simulink model "SinglePhaseInverter"  (R2021a)
settings: Solver=ode15s  StartTime=0.0  StopTime=0.1  FixedStep=1/fsw*PWM_Resolution  MaxStep=1/(4*fsw)  RelTol=1e-3  AbsTol=1e-3
PreLoadFcn:
  | Palam_SingleInverter;
undefined symbols (not defined in the file): DeadTime, fg, fsw, Initial_M, Kp, MaxDuty, MinDuty, Simple, Simscape, Ti, TimerCountMax, VinDC, VoutAC_rms
libraries: ee_lib x6, fl_lib x4, nesl_utility x4, slpidlib x1, eeGeneralControl x1, simulink x1
CloseFcn:
  | clear all
settings Model: Creator=ykamatan  LastModifiedBy=ykamatan
settings SolverCC: DaesscMode=Robust  ZeroCrossControl=EnableAll  ZeroCrossAlgorithm=Adaptive  AlgebraicLoopSolver=TrustRegion  ODENIntegrationMethod=ode1
settings DebuggingCC: SymbolicDimsDataTypeCodeGenerationDiagnostic=none  SFMachineParentedDataDiag=warning
settings SFSimCC: CustomCodeUndefinedFunction=UseInterfaceOnly
settings SimscapeCC: SimscapeLogType=local  SimscapeLogSimulationStatistics=on  SimscapeLogToSDI=on  SimscapeLogLimitData=off  SimscapeLogDataHistory=10000

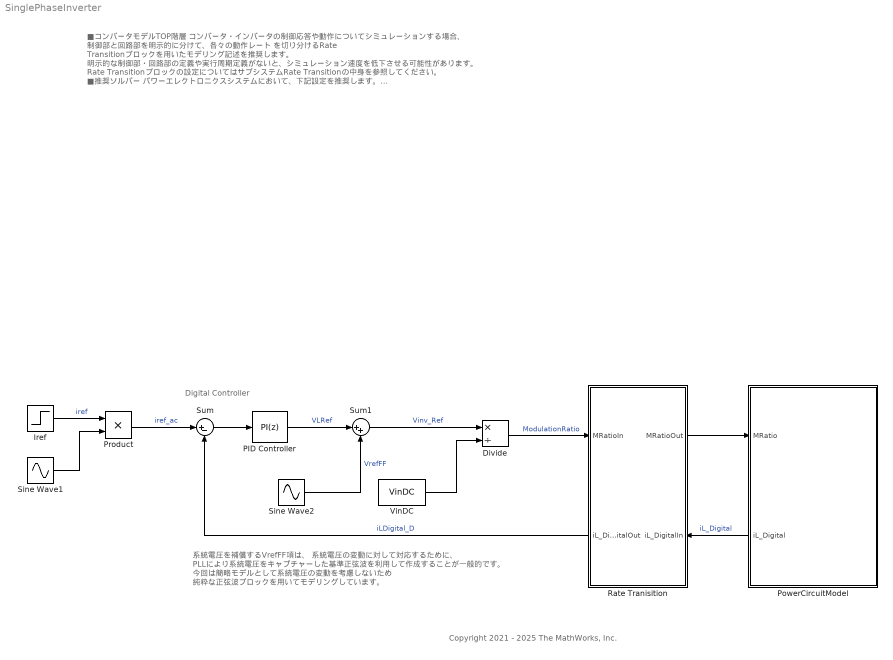
== system SinglePhaseInverter ==
  note: 系統電圧を補償するVrefFF項は、
      | 系統電圧の変動に対して対応するために、
      | PLLにより系統電圧をキャプチャーした基準正弦波を利用して作成することが一般的です。
      |
      | 今回は簡略モデルとして系統電圧の変動を考慮しないため
      | 純粋な正弦波ブロックを用いてモデリングしています。
  note: ■コンバータモデルTOP階層
      | コンバータ・インバータの制御応答や動作についてシミュレーションする場合、
      | 制御部と回路部を明示的に分けて、各々の動作レート を切り分けるRate Transitionブロックを用いたモデリング記述を推奨します。
      | 明示的な制御部・回路部の定義や実行周期定義がないと、シミュレーション速度を低下させる可能性があります。
      | Rate Transitionブロックの設定についてはサブシステムRate Transitionの中身を参照してください。
      |
      | ■推奨ソルバー
      | パワーエレクトロニクスシステムにおいて、下記設定を推奨します。
      | 最大ステップサイズに指定で用いている変数fswはスイッチング周波数です。
      | 最大ステップサイズを指定することで、可変ステップソルバがステップ数を長くしすぎることで、
      | Duｔｙパルス幅が指定周期に逐次更新されず、ずっとターンオンもしくはターンオンでシミュレーションが進行する現象が発生しなくなります。
  note: Digital Controller
  note: Copyright 2021 - 2025 The MathWorks, Inc.
  Divide : Product  Inputs=*/
  Iref : Step  Time=0.052  Before=5  After=10  SampleTime=1/fsw
  PID Controller : slpidlib/PID Controller  Controller=PI  Form=Parallel  TimeDomain=Discrete-time  UseExternalTs=off  SampleTime=1/fsw  IntegratorMethod=Forward Euler  FilterMethod=Forward Euler  ControllerParametersSource=internal  P=Kp  I=Ti  D=0  UseFilter=on  N=100  TunerSelectOption=Transfer Function Based (PID Tuner App)  InitialConditionSource=internal  InitialConditionForIntegrator=0  InitialConditionForFilter=0  DifferentiatorICPrevScaledInput=0  ExternalReset=none  TrackingMode=off  Kt=1  LimitOutput=off  SatLimitsSource=internal  UpperSaturationLimit=inf  LowerSaturationLimit=-inf  LinearizeAsGain=on  AntiWindupMode=none  Kb=1  POutMin=[]  POutMax=[]  IOutMin=[]  IOutMax=[]  DOutMin=[]  DOutMax=[]  NOutMin=[]  NOutMax=[]  SumOutMin=[]  SumOutMax=[]  SaturationOutMin=[]  SaturationOutMax=[]  PParamMin=[]  PParamMax=[]  IParamMin=[]  IParamMax=[]  DParamMin=[]  DParamMax=[]  NParamMin=[]  NParamMax=[]  KbParamMin=[]  KbParamMax=[]  KtParamMin=[]  KtParamMax=[]  KbOutMin=[]  KbOutMax=[]  KtOutMin=[]  KtOutMax=[]  IntegratorOutMin=[]  IntegratorOutMax=[]  FilterOutMin=[]  FilterOutMax=[]  SumI1OutMin=[]  SumI1OutMax=[]  SumI2OutMin=[]  SumI2OutMax=[]  SumI3OutMin=[]  SumI3OutMax=[]  SumI4OutMin=[]  SumI4OutMax=[]  SumDOutMin=[]  SumDOutMax=[]  DifferentiatorOutMin=[]  DifferentiatorOutMax=[]  FilterDiffOutCoefMin=[]  FilterDiffOutCoefMax=[]  ReciprocalOutMin=[]  ReciprocalOutMax=[]  SumDenOutMin=[]  SumDenOutMax=[]  SumNumOutMin=[]  SumNumOutMax=[]  DivideOutMin=[]  DivideOutMax=[]  UdiffTsProdOutMin=[]  UdiffTsProdOutMax=[]  NTsProdOutMin=[]  NTsProdOutMax=[]  UintegralTsProdOutMin=[]  UintegralTsProdOutMax=[]  UngainTsProdOutMin=[]  UngainTsProdOutMax=[]  IntegratorContinuousStateAttributes=''  IntegratorStateMustResolveToSignalObject=off  IntegratorRTWStateStorageClass=Auto  FilterContinuousStateAttributes=''  FilterStateMustResolveToSignalObject=off  FilterRTWStateStorageClass=Auto  ParallelPVariant=InternalParameters  IdealPVariant=Disabled  IVariant=InternalParameters  DVariant=Disabled  IntegratorVariant=Discrete  SatVariant=Disabled  AWVariant=Passthrough  PCopyVariant=Disabled  TRVariant=Disabled  FdbkBlocksVariant=Forward  IdealPFdbkVariant=Disabled  SatFdbkVariant=Disabled  DerivativeFilterVariant=Disabled  NVariant=Disabled  NCopyVariant=Disabled_SignalSpec  FilterICVariant=Disabled  IntegratorICVariant=InternalICs  ExternalResetVariant=Disabled  TRSumVariant=Passthrough  SumFdbkVariant=Disabled  SumVariant=Sum_PI  TsampFilterVariant=InternalTs  TsampNgainVariant=Passthrough  TsampIntegralVariant=Passthrough  ExternalSaturationOutDataTypeStr=Inherit: Same as second input
  PowerCircuitModel : Subsystem  VariantControl=Simulink+Simscape(Simple)
      settings: PortSchema="{\"entries\":[{\"content\":{\"sides\":[{\"content\":{\"connectorIds\":[\"In1\",\"Out1\"]},\"type\":\"ConnectorPlacement.EquallySpacedRectSide\",\"uuid\":\"190e0dea-1aa3-4142-a809-3b45efebbd06\"},{\"content\":{\"connectorIds\":[],\"side\":\"RIGHT\"},\"type\":\"ConnectorPlacement.EquallySpacedRectSide\",\"uuid\":\"b937fb0f-45e6-40ea-b2c8-56a8d22a3e17\"},{\"content\":{\"connectorIds\":[],\"side\":\"TOP\"},\"type\":\"ConnectorPlacement.EquallySpacedRectSide\",\"uuid\":\"78929584-fb1e-4361-895f-78605ee7c8f8\"}]},\"type\":\"ConnectorPlacement.EquallySpacedConnector\",\"uuid\":\"8246c905-c24d-44c3-959b-73866b615c12\"}],\"packageUris\":[\"http://schema.mathworks.com/mf0/Connector/R2020b\"],\"version\":\"1.0\"}"
  Product : Product
  "Rate Tranisition " : Subsystem
      settings: PortSchema="{\"entries\":[{\"content\":{\"sides\":[{\"content\":{\"connectorIds\":[\"In1\",\"Out2\"]},\"type\":\"ConnectorPlacement.EquallySpacedRectSide\",\"uuid\":\"82fdd683-de0b-47f1-9418-2e57132da0d0\"},{\"content\":{\"connectorIds\":[\"Out1\",\"In2\"],\"side\":\"RIGHT\"},\"type\":\"ConnectorPlacement.EquallySpacedRectSide\",\"uuid\":\"07812756-bbdf-4a3e-b825-c2cce10242a3\"},{\"content\":{\"connectorIds\":[],\"side\":\"TOP\"},\"type\":\"ConnectorPlacement.EquallySpacedRectSide\",\"uuid\":\"2a69d2b0-ad53-492d-9041-fc24e9d8466e\"}]},\"type\":\"ConnectorPlacement.EquallySpacedConnector\",\"uuid\":\"5e8493d4-adb1-45a0-b631-53482b8c22b1\"}],\"packageUris\":[\"http://schema.mathworks.com/mf0/Connector/R2020b\"],\"version\":\"1.0\"}"
  Sine Wave1 : Sin  Frequency=2*pi*fg  SampleTime=1/fsw
  Sine Wave2 : Sin  Amplitude=VoutAC_rms*sqrt(2)  Frequency=2*pi*fg  SampleTime=1/fsw
  Sum : Sum  Inputs=|+-
  Sum1 : Sum  Inputs=|++
  VinDC : Constant  Value=VinDC
  wires:
  PID Controller/1 -> Sum1/1  "VLRef"
  Sum/1 -> PID Controller/1
  Sum1/1 -> Divide/1  "Vinv_Ref"
  VinDC/1 -> Divide/2
  Product/1 -> Sum/1  "iref_ac"
  Divide/1 -> "Rate Tranisition "/1(MRatioIn)  "ModulationRatio"
  PowerCircuitModel/1(iL_Digital) -> "Rate Tranisition "/2(iL_DigitalIn)  "iL_Digital"
  "Rate Tranisition "/2(iL_DigitalOut) -> Sum/2  "iLDigital_D"
  "Rate Tranisition "/1(MRatioOut) -> PowerCircuitModel/1(MRatio)
  Iref/1 -> Product/1  "iref"
  Sine Wave1/1 -> Product/2
  Sine Wave2/1 -> Sum1/2  "VrefFF"

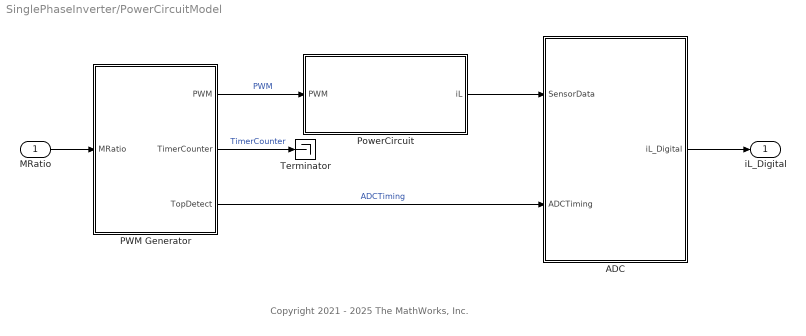
== system SinglePhaseInverter/PowerCircuitModel ==
  note: Copyright 2021 - 2025 The MathWorks, Inc.
  MRatio : Inport
  ADC : Subsystem
  PWM Generator : Subsystem
  PowerCircuit : Subsystem
  Terminator : Terminator
  iL_Digital : Outport
  wires:
  PowerCircuit/1(iL) -> ADC/1(SensorData)
  PWM Generator/1(PWM) -> PowerCircuit/1(PWM)  "PWM"
  PWM Generator/2(TimerCounter) -> Terminator/1  "TimerCounter"
  ADC/1(iL_Digital) -> iL_Digital/1
  MRatio/1 -> PWM Generator/1(MRatio)
  PWM Generator/3(TopDetect) -> ADC/2(ADCTiming)  "ADCTiming"

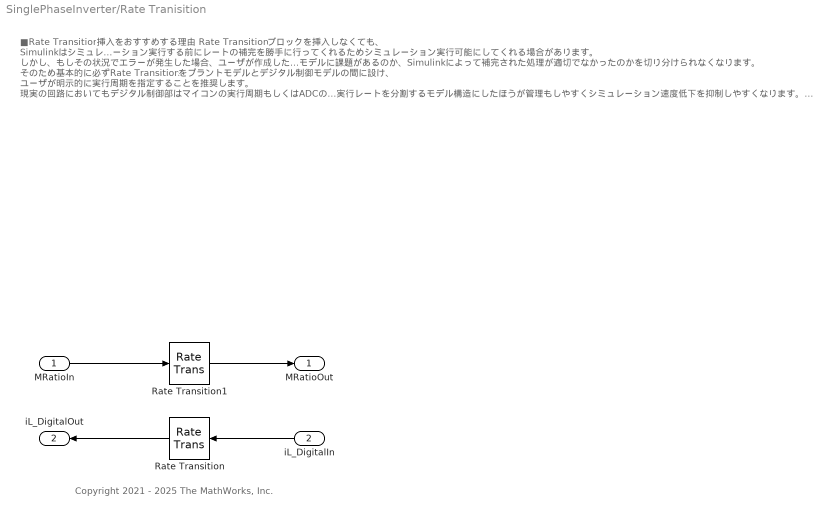
== system SinglePhaseInverter/Rate Tranisition  ==
  note: ■Rate Transition挿入をおすすめする理由
      | Rate Transitionブロックを挿入しなくても、
      | Simulinkはシミュレーション実行する前にレートの補完を勝手に行ってくれるためシミュレーション実行可能にしてくれる場合があります。
      |
      | しかし、もしその状況でエラーが発生した場合、ユーザが作成したモデルに課題があるのか、Simulinkによって補完された処理が適切でなかったのかを切り分けられなくなります。
      |
      | そのため基本的に必ずRate Transitionをプラントモデルとデジタル制御モデルの間に設け、
      | ユーザが明示的に実行周期を指定することを推奨します。
      |
      | 現実の回路においてもデジタル制御部はマイコンの実行周期もしくはADCの変換タイミングをトリガーに周期的に処理を行うため、明示的に実行レートを分割するモデル構造にしたほうが管理もしやすくシミュレーション速度低下を抑制しやすくなります。
      |
      | ■Rate Transitionのブロックパラメータ設定方法
      | ・データ転送中の整合性を確保
      | ・確定的にデータ転送を確保（最大遅延）
      | のチェックを入れておくことで、想定される最大のサンプリング遅れでサンプル値を取得するようにシミュレーションが動作します。これにより代数ループ警告も回避することができます。
      | ただし、このモデルのサンプリングはデジタルControllerモデルの実行周期(Tcnt = 1/fsw）分だけ必ずサンプリング値が遅れて伝搬されるため、制御ループの伝達関数を解析した際のむだ時間遅れは常に最悪の e^-sTcntとなることに注意が必要です。
  note: Copyright 2021 - 2025 The MathWorks, Inc.
  MRatioIn : Inport
  iL_DigitalIn : Inport  Port=2
  Rate Transition : RateTransition  OutPortSampleTime=1/fsw
  Rate Transition1 : RateTransition  InitialCondition=Initial_M
  MRatioOut : Outport
  iL_DigitalOut : Outport  Port=2
  wires:
  Rate Transition/1 -> iL_DigitalOut/1
  MRatioIn/1 -> Rate Transition1/1
  Rate Transition1/1 -> MRatioOut/1
  iL_DigitalIn/1 -> Rate Transition/1

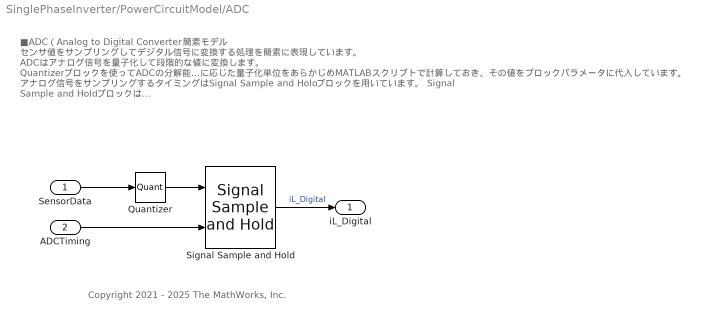
== system SinglePhaseInverter/PowerCircuitModel/ADC ==
  note: ■ADC（Analog to Digital Converter)簡素モデル
      | センサ値をサンプリングしてデジタル信号に変換する処理を簡素に表現しています。
      | ADCはアナログ信号を量子化して段階的な値に変換します。
      | Quantizerブロックを使ってADCの分解能に応じた量子化単位をあらかじめMATLABスクリプトで計算しておき、その値をブロックパラメータに代入しています。
      | アナログ信号をサンプリングするタイミングはSignal Sample and Holdブロックを用いています。
      | Signal Sample and Holdブロックは
      | Inにサンプリングしたい信号、Sにサンプリングタイミングを指定するパルス信号を入力することで、
      | そのタイミングでInの値をサンプリングし、それ以降次のパルスが入るまで値を保持します。
  note: Copyright 2021 - 2025 The MathWorks, Inc.
  SensorData : Inport
  ADCTiming : Inport  Port=2
  Quantizer : Quantizer  QuantizationInterval=QuantUnit
  Signal Sample and Hold : eeGeneralControl/Signal Sample and Hold  LabelModeActiveChoice=Discrete  x0=0  Ts=-1
      settings: SourceProductBaseCode=PS
  iL_Digital : Outport
  wires:
  Quantizer/1 -> Signal Sample and Hold/1
  Signal Sample and Hold/1 -> iL_Digital/1  "iL_Digital"
  ADCTiming/1 -> Signal Sample and Hold/2
  SensorData/1 -> Quantizer/1

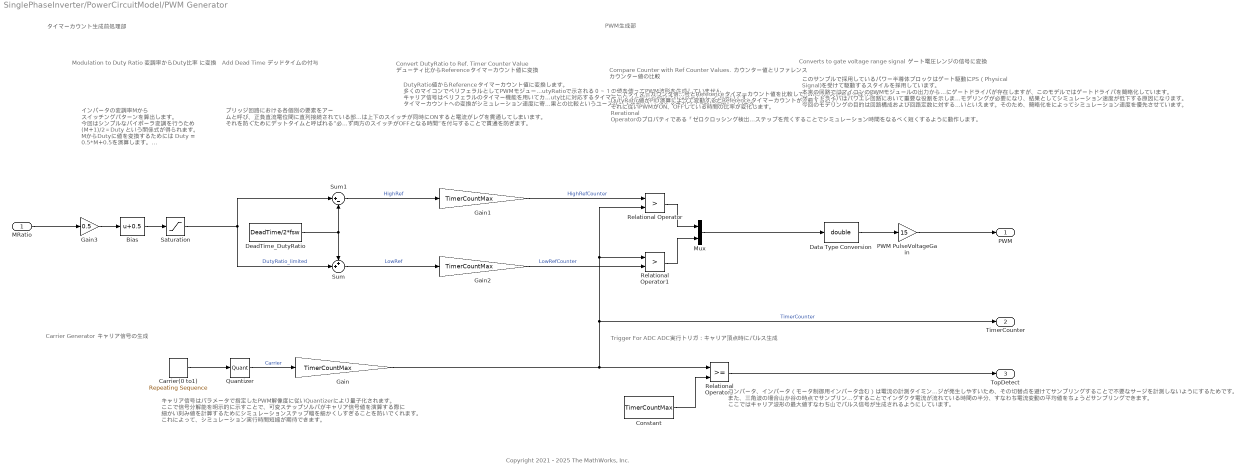
== system SinglePhaseInverter/PowerCircuitModel/PWM Generator ==
  note: PWM生成部
  note: タイマーカウント生成前処理部
  note: Modulation to
      | Duty Ratio
      |
      | 変調率からDuty比率
      | に変換
  note: キャリア信号はパラメータで指定したPWM解像度に従いQuantizerにより量子化されます。
      | ここで信号分解能を明示的に示すことで、可変ステップソルバがキャリア信号値を演算する際に
      | 細かい刻み値を計算するためにシミュレーションステップ幅を細かくしすぎることを防いでくれます。
      | これによって、シミュレーション実行時間短縮が期待できます。
  note: Converts to gate voltage range signal
      | ゲート電圧レンジの信号に変換
  note: Compare Counter with Ref Counter Values.
      | カウンター値とリファレンス カウンター値の比較
  note: Trigger For ADC
      | ADC実行トリガ：キャリア頂点時にパルス生成
  note: Convert DutyRatio to　Ref. Timer Counter Value
      | デューティ比からReferenceタイマーカウント値に変換
  note: Add Dead Time
      | デッドタイムの付与
  note: Carrier Generator
      | キャリア信号の生成
  note: Copyright 2021 - 2025 The MathWorks, Inc.
  note: ブリッジ回路における各個別の要素をアー ムと呼び、正負直流電位間に直列接続されている部分を上下一組でレグと呼びます。今回回路に用いているハーフブリッジ回路は単一のレグに相当します。レグを駆動する際には上下のスイッチが同時にONすると電流がレグを貫通してしまいます。
      | それを防ぐためにデットタイムと呼ばれる”必ず両方のスイッチがOFFとなる時間”を付与することで貫通を防ぎます。
  note: DutyRatio値からReferenceタイマーカウント値に変換します。
      | 多くのマイコンでペリフェラルとしてPWMモジュールが搭載されていますが、DutyRatioで示される０～１の値を使ってPWM波形を生成していません。
      |
      | キャリア信号はペリフェラルのタイマー機能を用いてカウントアップ・カウントダウンによって生成されるカウント値として指定されるので、Duty値もまた、Duty比に対応するタイマーカウント値に変換なければならないことが多いです。
      | タイマーカウントへの変換がシミュレーション速度に寄与する影響度は少ないですが、実機実験でのデバック結果との比較というユースケースを想定してタイマーカウント値に変換しています。
  note: ここでタイマーカウンタ信号とReferenceタイマーカウント値を比較してPWMパルス信号を生成します。
      |
      | DutyRatio値がPID演算によって変動するとReferenceタイマーカウントが変動するので、
      | それに従いPWMがON、OFFしている時間の比率が変化します。
      | Rerational Operatorのプロパティである「ゼロクロッシング検出を有効にする」を有効にすることで、可変ステップソルバは比較によって値が変動するタイミングで細かくステップを刻み、そうでない箇所ではタイムステップを荒くすることでシミュレーション時間をなるべく短くするように動作します。
  note: このサンプルで採用しているパワー半導体ブロックはゲート駆動にPS（Physical Signal)を受けて駆動するスタイルを採用しています。
      |
      | 本来の回路ではマイコンのPWMモジュールの出力からパワー半導体デバイスの間にゲートドライバが存在しますが、このモデルではゲートドライバを簡略化しています。
      |
      | ゲートドライバはパワエレ回路において重要な役割を示しますが、正確な挙動表現には細かいモデリングが必要になり、結果としてシミュレーション速度が低下する原因になります。
      | 今回のモデリングの目的は回路構成および回路定数に対する適切な制御則の導出であるため、目的に対してゲートドライバの詳細表現は影響度が少ないといえます。そのため、簡略化をによってシミュレーション速度を優先させています。
  note: コンバータ、インバータ（モータ制御用インバータ含む）は電流の計測タイミングをPWMキャリア信号と同期させることが多く、ノコギリ波の頂点、もしくは三角波の山か谷のタイミングでADCのサンプリングを行います。これはPWMパルス電圧が切り替わる瞬間は電流サージが発生しやすいため、その切替点を避けてサンプリングすることで不要なサージを計測しないようにするためです。
      | また、三角波の場合山か谷の時点でサンプリングすることでインダクタ電流が流れている時間の半分、すなわち電流変動の平均値をちょうどサンプリングできます。
      | ここではキャリア波形の最大値すなわち山でパルス信号が生成されるようにしています。
  note: インバータの変調率Mから
      | スイッチングパターンを算出します。
      |
      | 今回はシンプルなバイポーラ変調を行うため
      | (M+1)/2＝Duty
      | という関係式が得られます。
      | MからDutyに値を変換するためには
      | Duty = 0.5*M+0.5を演算します。
      |
      | 変調方式は回路構成によっても変わりますし、同じ回路で複数の変調方式を適応できるものもあるため、
      | 必要に応じて適切な演算を選択します。
      |
      | 最後にDutyの上限、加減を設定します
  MRatio : Inport
  Bias : Bias  Bias=0.5
  Carrier(0 to1) : simulink/Sources/Repeating Sequence  rep_seq_t=[0 1/fsw/2 1/fsw]  rep_seq_y=[1 0 1]
  Constant : Constant  Value=TimerCountMax  OutDataTypeStr=uint16
  Data Type Conversion : DataTypeConversion  OutDataTypeStr=double
  DeadTime_DutyRatio : Constant  Value=DeadTime/2*fsw  OutDataTypeStr=double
  Gain : Gain  Gain=TimerCountMax  OutDataTypeStr=double
  Gain1 : Gain  Gain=TimerCountMax
  Gain2 : Gain  Gain=TimerCountMax  OutDataTypeStr=double
  Gain3 : Gain  Gain=0.5
  Mux : Mux  Inputs=2
  PWM PulseVoltageGain : Gain  Gain=15
  Quantizer : Quantizer  QuantizationInterval=PWM_Resolution
  Relational Operator : RelationalOperator  Operator=>  OutDataTypeStr=boolean  RndMeth=Simplest  InputSameDT=on
  Relational Operator1 : RelationalOperator  Operator=>  OutDataTypeStr=boolean  RndMeth=Simplest  InputSameDT=on
  Relational Operator2 : RelationalOperator  OutDataTypeStr=boolean  RndMeth=Simplest
  Saturation : Saturate  UpperLimit=MaxDuty  LowerLimit=MinDuty
  Sum : Sum  Inputs=++|
  Sum1 : Sum  Inputs=|+-
  PWM : Outport
  TimerCounter : Outport  Port=2
  TopDetect : Outport  Port=3
  wires:
  Relational Operator1/1 -> Mux/2
  Data Type Conversion/1 -> PWM PulseVoltageGain/1
  Mux/1 -> Data Type Conversion/1
  Relational Operator/1 -> Mux/1
  PWM PulseVoltageGain/1 -> PWM/1
  Carrier(0 to1)/1 -> Quantizer/1
  Sum/1 -> Gain2/1  "LowRef"
  Saturation/1 -> Sum/2, Sum1/1  "DutyRatio_limited"
  DeadTime_DutyRatio/1 -> Sum1/2, Sum/1
  Constant/1 -> Relational Operator2/2
  Relational Operator2/1 -> TopDetect/1
  Quantizer/1 -> Gain/1  "Carrier"
  Gain/1 -> Relational Operator2/1, Relational Operator1/1, Relational Operator/2, TimerCounter/1  "TimerCounter"
  Gain1/1 -> Relational Operator/1  "HighRefCounter"
  Sum1/1 -> Gain1/1  "HighRef"
  Gain2/1 -> Relational Operator1/2  "LowRefCounter"
  MRatio/1 -> Gain3/1
  Bias/1 -> Saturation/1
  Gain3/1 -> Bias/1

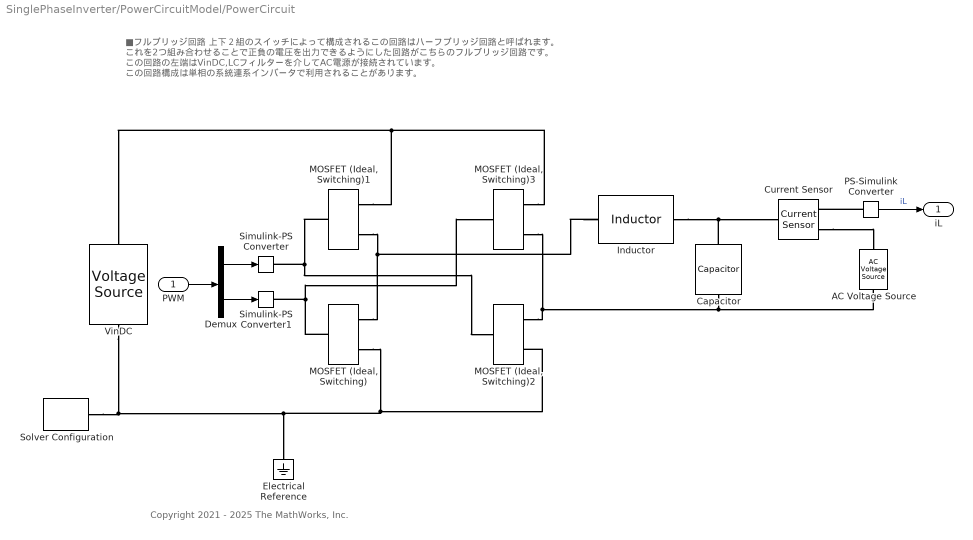
== system SinglePhaseInverter/PowerCircuitModel/PowerCircuit ==
  note: ■フルブリッジ回路
      | 上下２組のスイッチによって構成されるこの回路はハーフブリッジ回路と呼ばれます。
      | これを2つ組み合わせることで正負の電圧を出力できるようにした回路がこちらのフルブリッジ回路です。
      | この回路の左端はVinDC,LCフィルターを介してAC電源が接続されています。
      | この回路構成は単相の系統連系インバータで利用されることがあります。
  note: Copyright 2021 - 2025 The MathWorks, Inc.
  PWM : Inport
  AC Voltage Source : fl_lib/Electrical/Electrical Sources/AC Voltage Source  amp=VoutAC_rms*sqrt(2) V  shift=0 deg  frequency=fg Hz  omega=0 rad/s
  Capacitor : fl_lib/Electrical/Electrical Elements/Capacitor  c=10e-6 F  r=10e-3 Ohm  g=0 1/Ohm  i_specify=off  i_priority=None  i=0 A  i_nominal_specify=off  i_nominal_unit=A  i_nominal_value=1  v_specify=off  v_priority=None  v=0 V  v_nominal_specify=off  v_nominal_unit=V  v_nominal_value=1  vc_specify=off  vc_priority=High  vc=0 V  vc_nominal_specify=off  vc_nominal_unit=V  vc_nominal_value=1
  Current Sensor : fl_lib/Electrical/Electrical Sensors/Current Sensor
  Demux : Demux  Outputs=2
  Electrical Reference : fl_lib/Electrical/Electrical Elements/Electrical Reference
  Inductor : ee_lib/Passive/Inductor  l=L H  L_tol=20  enable_L_tol=0  tol_distribution=1  nSigma=4  r=0 Ohm  g=1e-9 1/Ohm  enable_operating_limits=0  operating_limit_action=2  max_working_current=1 A  power_rating=1 W  enable_faults=0  fault_action=1  lambdaPercent=50  k_faulted=0.9999  turnsShort=0  openCct=0  groundShort=0  groundShortG=0 1/Ohm  tau_fault=1e-3 s  enable_temporal_fault=0  t_fault=1 s  enable_behavioral_fault=0  max_permissible_voltage=100 V  n_fail_on_voltage=1  max_permissible_current=1 A  t_fail_on_current=1 s  i_L_specify=off  i_L_priority=High  i_L=0 A  i_L_nominal_specify=off  i_L_nominal_unit=A  i_L_nominal_value=1
  MOSFET (Ideal, Switching){,1..3} (4 alike) : ee_lib/Semiconductors & Converters/MOSFET (Ideal, Switching)  Rds=0.01 Ohm  Goff=1e-6 1/Ohm  Vth=2 V  diode_param=2  diode_Vf=0.8 V  diode_Ron=0.001 Ohm  diode_Goff=1e-5 1/Ohm  diode_C=50e-9 F  diode_iRM=-235 A  diode_iF=300 A  diode_idot=-50 A/us  diode_trr_param=1  diode_trr_factor=3  diode_trr=15 us  diode_Qrr=1500 s*uA  thermal_loss_option=ee.enum.converters.thermalLossOption.constantvalues  Von_data=[0, 1.1, 1.3, 1.45, 1.75, 2.25, 2.7; 0, 1, 1.15, 1.35, 1.7, 2.35, 3] V  Eon_data=[0, .29, 1.43, 2.86, 5.71, 13.14, 22.86; 0, .57, 2.63, 5.14, 10.29, 20.57, 30.29] * 1e-3 J  Eoff_data=[0, .21, 1.07, 2.14, 4.29, 9.86, 17.14; 0, .43, 1.97, 3.86, 7.71, 15.43, 22.71] * 1e-3 J  Tj=[298.15, 398.15] K  Iout_data=[0, 10, 50, 100, 200, 400, 600] A  Eon_scalar=22.86e-3 J  Eoff_scalar=17.14e-3 J  Voff=300 V  Iout_scalar=600 A  diodeModelType=ee.enum.converters.diodeModelType.pwl  diode_IfMat=[.07, .12, .19, 1.75, 4.24, 7.32, 11.2; .16, .3, .72, 2.14, 4.02, 6.35, 9.12] A  diode_TjVec=[25, 125] degC  diode_VfVec=[.5, .7, .9, 1.3, 1.7, 2.1, 2.5] V  thermal_network_parameterization=ee.enum.thermalNetworkTopology.external  Rth=[.03, .2] K/W  Rth_Foster=[.03, .2] K/W  thermal_mass_parameterization=ee.enum.thermalNetwork.timeconstant  thermal_mass=[3, 25] J/K  thermal_mass_Foster=[33, 50] J/K  thermal_time_constant=[.1, 5] s  thermal_time_constant_Foster=[1, 10] s  thermal_mass_initial_temperatures=[25, 25] degC  junction_thermal_mass=0.1 J/K  vT_specify=off  vT_priority=None  vT=0 V  vT_nominal_specify=off  vT_nominal_unit=V  vT_nominal_value=1  Qj_specify=off  Qj_priority=None  Qj=0 W  Qj_nominal_specify=off  Qj_nominal_unit=W  Qj_nominal_value=1  junction_temperature_specify=off  junction_temperature_priority=None  junction_temperature=25 degC  junction_temperature_nominal_specify=off  junction_temperature_nominal_unit=degC  junction_temperature_nominal_value=1
  PS-Simulink Converter : nesl_utility/PS-Simulink Converter  PhysicalDomain=network_engine_domain  SubClassName=ps_output  LeftPortType=input  RightPortType=output  PseudoPeriodic=off  Frequencies=[]  Unit=inherit  AffineConversion=off
      settings: SourceProductBaseCode=PW,SS
  Simulink-PS Converter : nesl_utility/Simulink-PS Converter  PhysicalDomain=network_engine_domain  SubClassName=ps_input  LeftPortType=input  RightPortType=output  PseudoPeriodic=off  Frequencies=[]  NoiseDistribution=none  NoiseParameters=[]  Unit=1  AffineConversion=off  FilteringAndDerivatives=provide  SimscapeFilterOrder=1  InputFilterTimeConstant=0.001  UdotUserProvided=0
      settings: SourceProductBaseCode=PW,SS
  Simulink-PS Converter1 : nesl_utility/Simulink-PS Converter  PhysicalDomain=network_engine_domain  SubClassName=ps_input  LeftPortType=input  RightPortType=output  PseudoPeriodic=off  Frequencies=[]  NoiseDistribution=none  NoiseParameters=[]  Unit=1  AffineConversion=off  FilteringAndDerivatives=provide  SimscapeFilterOrder=1  InputFilterTimeConstant=0.001  UdotUserProvided=0
      settings: SourceProductBaseCode=PW,SS
  Solver Configuration : nesl_utility/Solver Configuration  PhysicalDomain=network_engine_domain  SubClassName=solver  LeftPortType=input  RightPortType=generic  Tones=[]  Harmonics=[]  SimulateNoise=off  Profile=off  UseLocalSampling=off  EnableSwitchedLinearOptims=on  FrequencyDomain=off  UseCCode=off  RelTol=0.001  AbsTol=1e-06  MinStep=1e-09  ToWorkspace=off  RevertToSquareIcSolve=off  NumHomotopyIterations=100  PhasorMode=off  PhasorModeNumHarmonics=1  DoDC=off  ResidualTolerance=1e-09  UseLocalSolver=off  LocalSolverChoice=NE_BACKWARD_EULER_ADVANCER  LocalSolverSampleTime=0.001  DoFixedCost=off  MaxNonlinIter=3  MaxModeIter=2  ComputeImpulses=off  ImpulseIterations=2  LinearAlgebra=auto  EquationFormulation=NE_TIME_EF  DelaysMemoryBudget=1024  AutomaticFiltering=on  FilteringTimeConstant=0.001  PartitionStorageMethod=AS_NEEDED  PartitionMemoryBudget=1024  PartitionMethod=ROBUST
      settings: SourceProductBaseCode=PW,SS
  VinDC : ee_lib/Sources/Voltage Source  dc_voltage=VinDC V  ac_voltage=0 V  ac_shift=0 rad  ac_frequency=0 Hz  noise_mode=0  PSD=0 V^2/Hz  repeatability=1  auto_seed=3499211588  user_seed=0  sample_time=1e-3 s  i_specify=off  i_priority=None  i=0 A  i_nominal_specify=off  i_nominal_unit=A  i_nominal_value=1  v_specify=off  v_priority=None  v=0 V  v_nominal_specify=off  v_nominal_unit=V  v_nominal_value=1
      settings: AttributesFormatString=DCV = %<dc_voltage>[V]
  iL : Outport
  wires:
  Demux/1 -> Simulink-PS Converter/1
  Demux/2 -> Simulink-PS Converter1/1
  PWM/1 -> Demux/1
  PS-Simulink Converter/1 -> iL/1  "iL"
  connections:
  "MOSFET (Ideal, Switching)"/RConn1 -- "MOSFET (Ideal, Switching)1"/RConn2 -- Inductor/LConn1
  "MOSFET (Ideal, Switching)1"/RConn1 -- VinDC/LConn1 -- "MOSFET (Ideal, Switching)3"/RConn1
  PS-Simulink Converter/LConn1 -- Current Sensor/RConn1
  "MOSFET (Ideal, Switching)1"/LConn1 -- Simulink-PS Converter/RConn1 -- "MOSFET (Ideal, Switching)2"/LConn1
  Solver Configuration/RConn1 -- VinDC/RConn1 -- "MOSFET (Ideal, Switching)2"/RConn2 -- "MOSFET (Ideal, Switching)"/RConn2 -- Electrical Reference/LConn1
  "MOSFET (Ideal, Switching)"/LConn1 -- "MOSFET (Ideal, Switching)3"/LConn1 -- Simulink-PS Converter1/RConn1
  Inductor/RConn1 -- Capacitor/LConn1 -- Current Sensor/LConn1
  Current Sensor/RConn2 -- AC Voltage Source/LConn1
  "MOSFET (Ideal, Switching)3"/RConn2 -- "MOSFET (Ideal, Switching)2"/RConn1 -- AC Voltage Source/RConn1 -- Capacitor/RConn1
